simulink model "FM"  (R2019b)
settings: Solver=VariableStepAuto  StartTime=0.0  StopTime=10.0  RelTol=1e-3
libraries: commanapbnd3 x2
settings Model: Creator=Win 10  LastModifiedBy=thuma

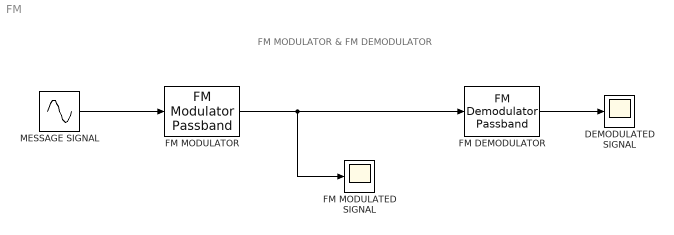
== system FM ==
  note: FM MODULATOR & FM DEMODULATOR
  DEMODULATED SIGNAL : Scope
  "FM DEMODULATOR " : commanapbnd3/FM Demodulator Passband  Fc=300  Ph=0  Kc=50  Ho=100
      settings: SourceProductName=Communications Toolbox  SourceProductBaseCode=CM
  FM MODULATED SIGNAL : Scope
  FM MODULATOR : commanapbnd3/FM Modulator Passband  Fc=25  Ph=0  Kc=10
      settings: SourceProductName=Communications Toolbox  SourceProductBaseCode=CM
  MESSAGE SIGNAL : Sin  Frequency=2*pi*1  SampleTime=0.001
  wires:
  MESSAGE SIGNAL/1 -> FM MODULATOR/1
  FM MODULATOR/1 -> "FM DEMODULATOR "/1, FM MODULATED SIGNAL/1
  "FM DEMODULATOR "/1 -> DEMODULATED SIGNAL/1
